simulink model "Path_Finder"  (R2024b)
settings: Solver=VariableStepAuto  StartTime=0.0  StopTime=200  RelTol=1e-3
model workspace (MAT data in the model file):
  Drag_Constants = 1
  mass = [5.51 5.51 5.51 1 1 1]
  mass_6a = [5 5 5 1 1 1]
libraries: simulink x1
settings Model: Creator=zenyn  LastModifiedBy=zenyn
settings DebuggingCC: UnderSpecifiedDimensionMsg=warning

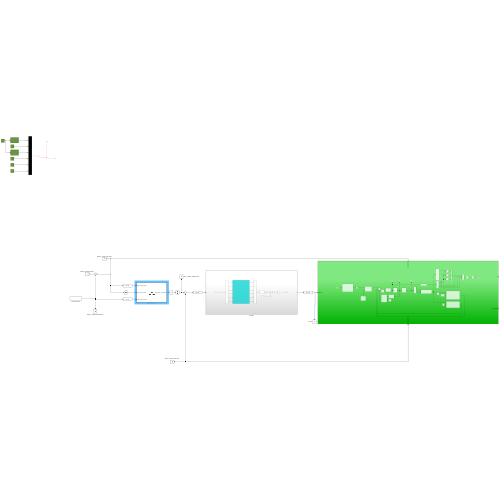
[thumbnail: Simulink's stored preview of the top-level diagram]
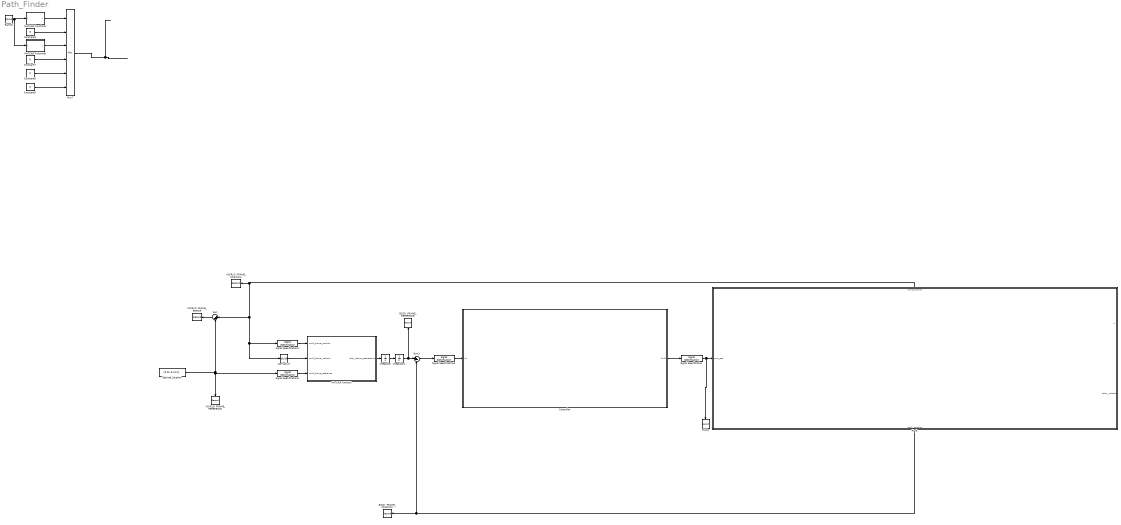
== system Path_Finder ==
  BODY_FRAME_POSITION : Record  FileSettingsInternal="{\"entries\":[{\"content\":{\"excelSettings\":{\"content\":{},\"type\":\"Streamout.ExcelSettings\"}},\"type\":\"Streamout.FileSettingStorage\",\"uuid\":\"\"}],\"packageUris\":[\"http:\\/\\/schema.mathworks.com\\/mf0\\/streamout_blocks\\/R2020a\"],\"version\":\"1.0\"}"  Layout=[1 1]  SignalsInternal="{\"entries\":[{\"content\":{},\"type\":\"RecordBlkView.InputSignals\",\"uuid\":\"\"}],\"packageUris\":[\"http:\\/\\/schema.mathworks.com\\/mf0\\/streamout_blocks\\/R2020a\"],\"version\":\"1.0\"}"  VisualizationBindings="{\"sparklinesplugin\":{\"info\":[{\"bindingParametersList\":[],\"subplotID\":1}]}}"
  BODY_FRAME_REFERENCE : Record  FileSettingsInternal="{\"entries\":[{\"content\":{\"excelSettings\":{\"content\":{},\"type\":\"Streamout.ExcelSettings\"}},\"type\":\"Streamout.FileSettingStorage\",\"uuid\":\"\"}],\"packageUris\":[\"http:\\/\\/schema.mathworks.com\\/mf0\\/streamout_blocks\\/R2020a\"],\"version\":\"1.0\"}"  SignalsInternal="{\"entries\":[{\"content\":{},\"type\":\"RecordBlkView.InputSignals\",\"uuid\":\"\"}],\"packageUris\":[\"http:\\/\\/schema.mathworks.com\\/mf0\\/streamout_blocks\\/R2020a\"],\"version\":\"1.0\"}"  VisualizationBindings="{\"sparklinesplugin\":{\"info\":[{\"bindingParametersList\":[],\"subplotID\":1}]}}"
  Constant{6..9} (4 alike) : Constant  Value=0
  Controller : Subsystem
  Derivative : Derivative
  Desired Location : Constant  Value=[0 20 -5 0 0 1]
  Integrator : Integrator
  Integrator1 : Integrator
  MATLAB Function : MATLAB Function  TreatAsAtomicUnit=on
  MATLAB Function6 : MATLAB Function  TreatAsAtomicUnit=on
  MATLAB Function8 : MATLAB Function  TreatAsAtomicUnit=on
  Mux7 : Mux  Inputs=6
  PWMs : Record  FileSettingsInternal="{\"entries\":[{\"content\":{\"excelSettings\":{\"content\":{},\"type\":\"Streamout.ExcelSettings\"}},\"type\":\"Streamout.FileSettingStorage\",\"uuid\":\"\"}],\"packageUris\":[\"http:\\/\\/schema.mathworks.com\\/mf0\\/streamout_blocks\\/R2020a\"],\"version\":\"1.0\"}"  Layout=[1 1]  SignalsInternal="{\"entries\":[{\"content\":{},\"type\":\"RecordBlkView.InputSignals\",\"uuid\":\"\"}],\"packageUris\":[\"http:\\/\\/schema.mathworks.com\\/mf0\\/streamout_blocks\\/R2020a\"],\"version\":\"1.0\"}"  VisualizationBindings="{\"sparklinesplugin\":{\"info\":[{\"bindingParametersList\":[],\"subplotID\":1}]}}"
  Plant : Subsystem
      settings: PortSchema="{\"entries\":[{\"content\":{\"sides\":[{\"content\":{\"connectorIds\":[\"In1\"]},\"type\":\"ConnectorPlacement.EquallySpacedRectSide\",\"uuid\":\"dd5f5d00-f9c2-4307-bbb7-eccecd8688a5\"},{\"content\":{\"connectorIds\":[\"Out1\",\"Out2\"],\"side\":\"RIGHT\"},\"type\":\"ConnectorPlacement.EquallySpacedRectSide\",\"uuid\":\"260bc773-df58-4a30-8a2b-ed16ecf586eb\"},{\"content\":{\"connectorIds\":[\"Out4\"],\"side\":\"TOP\"},\"type\":\"ConnectorPlacement.EquallySpacedRectSide\",\"uuid\":\"8636c4da-abe4-4bf1-a8cd-e88e3163142a\"},{\"content\":{\"connectorIds\":[\"Out3\"],\"side\":\"BOTTOM\"},\"type\":\"ConnectorPlacement.EquallySpacedRectSide\",\"uuid\":\"d94fc4d4-7054-443b-b127-f4054aef1378\"}]},\"type\":\"ConnectorPlacement.EquallySpacedConnector\",\"uuid\":\"031b742f-18b9-426f-a877-fafb44a51bf1\"}],\"packageUris\":[\"http://schema.mathworks.com/mf0/Connector/R2020b\"],\"version\":\"1.0\"}"
  Ramp2 : simulink/Sources/Ramp  slope=1  start=0  InitialOutput=0
  Signal Specification : SignalSpecification  Dimensions=[ 1 8]
  Signal Specification1 : SignalSpecification  Dimensions=[ 1 6]
  Signal Specification2 : SignalSpecification  Dimensions=[1 6]
  Signal Specification3 : SignalSpecification  Dimensions=[1 6]
  Sum : Sum  Inputs=|+-
  Sum1 : Sum  Inputs=|+-
  WORLD_FRAME_ERROR : Record  FileSettingsInternal="{\"entries\":[{\"content\":{\"excelSettings\":{\"content\":{},\"type\":\"Streamout.ExcelSettings\"}},\"type\":\"Streamout.FileSettingStorage\",\"uuid\":\"\"}],\"packageUris\":[\"http:\\/\\/schema.mathworks.com\\/mf0\\/streamout_blocks\\/R2020a\"],\"version\":\"1.0\"}"  Layout=[1 1]  SignalsInternal="{\"entries\":[{\"content\":{},\"type\":\"RecordBlkView.InputSignals\",\"uuid\":\"\"}],\"packageUris\":[\"http:\\/\\/schema.mathworks.com\\/mf0\\/streamout_blocks\\/R2020a\"],\"version\":\"1.0\"}"  VisualizationBindings="{\"sparklinesplugin\":{\"info\":[{\"bindingParametersList\":[],\"subplotID\":1}]}}"
  WORLD_FRAME_POSITION : Record  FileSettingsInternal="{\"entries\":[{\"content\":{\"excelSettings\":{\"content\":{},\"type\":\"Streamout.ExcelSettings\"}},\"type\":\"Streamout.FileSettingStorage\",\"uuid\":\"\"}],\"packageUris\":[\"http:\\/\\/schema.mathworks.com\\/mf0\\/streamout_blocks\\/R2020a\"],\"version\":\"1.0\"}"  Layout=[1 1]  SignalsInternal="{\"entries\":[{\"content\":{},\"type\":\"RecordBlkView.InputSignals\",\"uuid\":\"\"}],\"packageUris\":[\"http:\\/\\/schema.mathworks.com\\/mf0\\/streamout_blocks\\/R2020a\"],\"version\":\"1.0\"}"  VisualizationBindings="{\"sparklinesplugin\":{\"info\":[{\"bindingParametersList\":[],\"subplotID\":1}]}}"
  WORLD_FRAME_REFERENCE : Record  FileSettingsInternal="{\"entries\":[{\"content\":{\"excelSettings\":{\"content\":{},\"type\":\"Streamout.ExcelSettings\"}},\"type\":\"Streamout.FileSettingStorage\",\"uuid\":\"\"}],\"packageUris\":[\"http:\\/\\/schema.mathworks.com\\/mf0\\/streamout_blocks\\/R2020a\"],\"version\":\"1.0\"}"  Layout=[1 1]  SignalsInternal="{\"entries\":[{\"content\":{\"signals\":[{\"content\":{\"blockPath\":[],\"dimensions\":[1,6],\"domain\":\"\",\"hasChildren\":true,\"lineColor\":\"#edb120\",\"lineWidth\":2,\"port\":1,\"sid\":[\"\"],\"signalID\":1,\"signalName\":\"Plant:3\"},\"type\":\"RecordBlkView.Signal\",\"uuid\":\"\"},{\"content\":{\"blockPath\":[],\"channel\":[1,1],\"dimensions\":[1,6],\"domain\":\"\",\"lineColor\":\"#7e2f8e\",\"lineWidth\":2,\"parentID\":1,\"port\":1,\"sid\":[\"\"],\"signalID\":2,\"signalName\":\"Plant:3\"},\"type\":\"RecordBlkView.Signal\",\"uuid\":\"\"},{\"content\":{\"blockPath\":[],\"dimensions\":[1,6],\"domain\":\"\",\"hasChildren\":true,\"lineColor\":\"#77ac30\",\"lineWidth\":2,\"port\":1,\"sid\":[\"\"],\"signalID\":3,\"signalName\":\"Integrator1\"},\"type\":\"RecordBlkView.Signal\",\"uuid\":\"\"},{\"content\":{\"blockPath\":[],\"channel\":[1,1],\"dimensions\":[1,6],\"domain\":\"\",\"lineColor\":\"#0072bd\",\"lineWidth\":2,\"parentID\":3,\"port\":1,\"sid\":[\"\"],\"signalID\":4,\"signalName\":\"Integrator1\"},\"type\":\"RecordBlkView.Signal\",\"uuid\":\"\"},{\"content\":{\"blockPath\":[],\"dimensions\":[1,8],\"domain\":\"\",\"hasChildren\":true,\"lineColor\":\"#a2142f\",\"lineWidth\":2,\"port\":1,\"sid\":[\"\"],\"signalID\":5,\"signalName\":\"Signal Specification\"},\"type\":\"RecordBlkView.Signal\",\"uuid\":\"\"},{\"content\":{\"blockPath\":[],\"channel\":[1,1],\"dimensions\":[1,8],\"domain\":\"\",\"lineColor\":\"#139fff\",\"lineWidth\":2,\"parentID\":5,\"port\":1,\"sid\":[\"\"],\"signalID\":6,\"signalName\":\"Signal Specification\"},\"type\":\"RecordBlkView.Signal\",\"uuid\":\"\"},{\"content\":{\"blockPath\":[],\"dimensions\":[6],\"domain\":\"\",\"hasChildren\":true,\"lineColor\":\"#ff6929\",\"lineWidth\":2,\"port\":1,\"sid\":[\"\"],\"signalID\":7,\"signalName\":\"Sum\"},\"type\":\"RecordBlkView.Signal\",\"uuid\":\"\"},{\"content\":{\"blockPath\":[],\"channel\":[1],\"dimensions\":[6],\"domain\":\"\",\"lineColor\":\"#edb120\",\"lineWidth\":2,\"parentID\":7,\"port\":1,\"sid\":[\"\"],\"signalID\":8,\"signalName\":\"Sum\"},\"type\":\"RecordBlkView.Signal\",\"uuid\":\"\"},{\"content\":{\"blockPath\":[],\"dimensions\":[6],\"domain\":\"\",\"hasChildren\":true,\"lineColor\":\"#64d413\",\"lineWidth\":2,\"port\":1,\"sid\":[\"\"],\"signalID\":9,\"signalName\":\"Plant:4\"},\"type\":\"RecordBlkView.Signal\",\"uuid\":\"\"},{\"content\":{\"blockPath\":[],\"channel\":[1],\"dimensions\":[6],\"domain\":\"\",\"lineColor\":\"#ff13a6\",\"lineWidth\":2,\"parentID\":9,\"port\":1,\"sid\":[\"\"],\"signalID\":10,\"signalName\":\"Plant:4\"},\"type\":\"RecordBlkView.Signal\",\"uuid\":\"\"},{\"content\":{\"blockPath\":[],\"dimensions\":[1,6],\"domain\":\"\",\"hasChildren\":true,\"lineColor\":\"#fe330a\",\"lineWidth\":2,\"port\":1,\"sid\":[\"\"],\"signalID\":11},\"type\":\"RecordBlkView.Signal\",\"uuid\":\"\"},{\"content\":{\"blockPath\":[],\"channel\":[1,1],\"dimensions\":[1,6],\"domain\":\"\",\"lineColor\":\"#22b573\",\"lineWidth\":2,\"parentID\":11,\"port\":1,\"sid\":[\"\"],\"signalID\":12},\"type\":\"RecordBlkView.Signal\",\"uuid\":\"\"},{\"content\":{\"blockPath\":[],\"dimensions\":[6],\"domain\":\"\",\"hasChildren\":true,\"lineColor\":\"#0072bd\",\"lineWidth\":2,\"port\":1,\"sid\":[\"\"],\"signalID\":13,\"signalName\":\"Desired Location\"},\"type\":\"RecordBlkView.Signal\",\"uuid\":\"\"},{\"content\":{\"blockPath\":[],\"channel\":[1],\"dimensions\":[6],\"domain\":\"\",\"lineColor\":\"#d95319\",\"lineWidth\":2,\"parentID\":13,\"port\":1,\"sid\":[\"\"],\"signalID\":14,\"signalName\":\"Desired Location\"},\"type\":\"RecordBlkView.Signal\",\"uuid\":\"\"},{\"content\":{\"blockPath\":[],\"channel\":[2],\"dimensions\":[6],\"domain\":\"\",\"lineColor\":\"#a2142f\",\"lineWidth\":2,\"parentID\":7,\"port\":1,\"sid\":[\"\"],\"signalID\":15,\"signalName\":\"Sum\"},\"type\":\"RecordBlkView.Signal\",\"uuid\":\"\"},{\"content\":{\"blockPath\":[],\"channel\":[3],\"dimensions\":[6],\"domain\":\"\",\"lineColor\":\"#139fff\",\"lineWidth\":2,\"parentID\":7,\"port\":1,\"sid\":[\"\"],\"signalID\":16,\"signalName\":\"Sum\"},\"type\":\"RecordBlkView.Signal\",\"uuid\":\"\"},{\"content\":{\"blockPath\":[],\"channel\":[4],\"dimensions\":[6],\"domain\":\"\",\"lineColor\":\"#ff6929\",\"lineWidth\":2,\"parentID\":7,\"port\":1,\"sid\":[\"\"],\"signalID\":17,\"signalName\":\"Sum\"},\"type\":\"RecordBlkView.Signal\",\"uuid\":\"\"},{\"content\":{\"blockPath\":[],\"channel\":[5],\"dimensions\":[6],\"domain\":\"\",\"lineColor\":\"#b746ff\",\"lineWidth\":2,\"parentID\":7,\"port\":1,\"sid\":[\"\"],\"signalID\":18,\"signalName\":\"Sum\"},\"type\":\"RecordBlkView.Signal\",\"uuid\":\"\"},{\"content\":{\"blockPath\":[],\"channel\":[6],\"dimensions\":[6],\"domain\":\"\",\"lineColor\":\"#64d413\",\"lineWidth\":2,\"parentID\":7,\"port\":1,\"sid\":[\"\"],\"signalID\":19,\"signalName\":\"Sum\"},\"type\":\"RecordBlkView.Signal\",\"uuid\":\"\"},{\"content\":{\"blockPath\":[],\"channel\":[1,2],\"dimensions\":[1,6],\"domain\":\"\",\"lineColor\":\"#139fff\",\"lineWidth\":2,\"parentID\":3,\"port\":1,\"sid\":[\"\"],\"signalID\":20,\"signalName\":\"Integrator1\"},\"type\":\"RecordBlkView.Signal\",\"uuid\":\"\"},{\"content\":{\"blockPath\":[],\"channel\":[1,3],\"dimensions\":[1,6],\"domain\":\"\",\"lineColor\":\"#ff6929\",\"lineWidth\":2,\"parentID\":3,\"port\":1,\"sid\":[\"\"],\"signalID\":21,\"signalName\":\"Integrator1\"},\"type\":\"RecordBlkView.Signal\",\"uuid\":\"\"},{\"content\":{\"blockPath\":[],\"channel\":[1,4],\"dimensions\":[1,6],\"domain\":\"\",\"lineColor\":\"#b746ff\",\"lineWidth\":2,\"parentID\":3,\"port\":1,\"sid\":[\"\"],\"signalID\":22,\"signalName\":\"Integrator1\"},\"type\":\"RecordBlkView.Signal\",\"uuid\":\"\"},{\"content\":{\"blockPath\":[],\"channel\":[1,5],\"dimensions\":[1,6],\"domain\":\"\",\"lineColor\":\"#64d413\",\"lineWidth\":2,\"parentID\":3,\"port\":1,\"sid\":[\"\"],\"signalID\":23,\"signalName\":\"Integrator1\"},\"type\":\"RecordBlkView.Signal\",\"uuid\":\"\"},{\"content\":{\"blockPath\":[],\"channel\":[1,6],\"dimensions\":[1,6],\"domain\":\"\",\"lineColor\":\"#ff13a6\",\"lineWidth\":2,\"parentID\":3,\"port\":1,\"sid\":[\"\"],\"signalID\":24,\"signalName\":\"Integrator1\"},\"type\":\"RecordBlkView.Signal\",\"uuid\":\"\"}]},\"type\":\"RecordBlkView.InputSignals\",\"uuid\":\"\"}],\"packageUris\":[\"http:\\/\\/schema.mathworks.com\\/mf0\\/streamout_blocks\\/R2020a\"],\"version\":\"1.0\"}"  VisualizationBindings="{\"sparklinesplugin\":{\"info\":[{\"bindingParametersList\":[],\"subplotID\":1}]}}"
  wires:
  Plant/4(world_position) -> Sum/1, Derivative/1, Signal Specification1/1, WORLD_FRAME_POSITION/1
  MATLAB Function8/1(y) -> Mux7/3
  Mux7/1 -> ?
  Constant6/1 -> Mux7/2
  Ramp2/1 -> MATLAB Function6/1(t), MATLAB Function8/1(t)
  Constant8/1 -> Mux7/5
  Constant9/1 -> Mux7/6
  MATLAB Function6/1(y) -> Mux7/1
  Constant7/1 -> Mux7/4
  Desired Location/1 -> Sum/2, Signal Specification2/1, WORLD_FRAME_REFERENCE/1
  Controller/1(Out1) -> Signal Specification/1
  Signal Specification/1 -> PWMs/1, Plant/1(pwm_set)
  Plant/3(body_position) -> Sum1/2, BODY_FRAME_POSITION/1
  Signal Specification3/1 -> Controller/1(In1)
  Sum1/1 -> Signal Specification3/1
  Signal Specification1/1 -> MATLAB Function/1(world_frame_position)
  Signal Specification2/1 -> MATLAB Function/3(world_frame_reference)
  MATLAB Function/1(body_frame_acceleration) -> Integrator/1
  Integrator/1 -> Integrator1/1
  Sum/1 -> WORLD_FRAME_ERROR/1
  Derivative/1 -> MATLAB Function/2(world_frame_velocity)
  Integrator1/1 -> BODY_FRAME_REFERENCE/1, Sum1/1

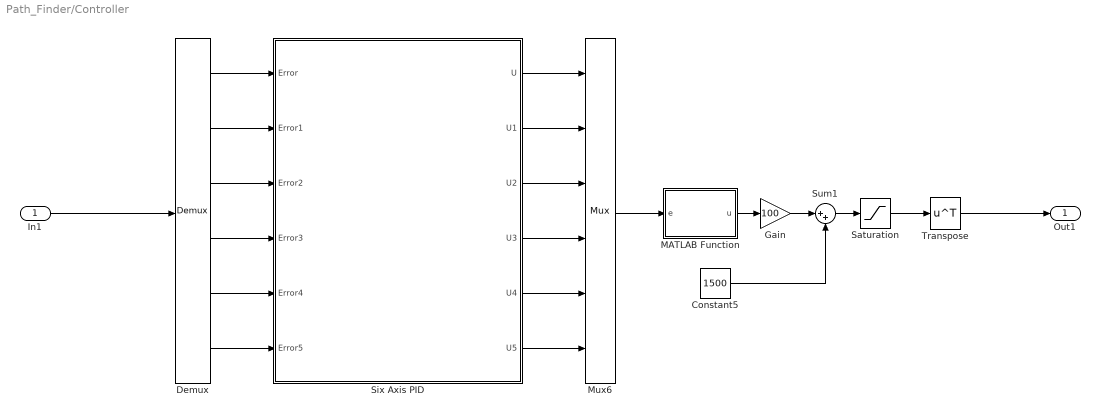
== system Path_Finder/Controller ==
  In1 : Inport
  Constant5 : Constant  Value=1500
  Demux : Demux  Outputs=6
  Gain : Gain  Gain=100
  MATLAB Function : MATLAB Function  TreatAsAtomicUnit=on
  Mux6 : Mux  Inputs=6
  Saturation : Saturate  UpperLimit=1900  LowerLimit=1100
  Six Axis PID : Subsystem
  Sum1 : Sum  Inputs=|++
  Transpose : Math  Operator=transpose
  Out1 : Outport
  wires:
  Saturation/1 -> Transpose/1
  Sum1/1 -> Saturation/1
  Demux/6 -> Six Axis PID/6(Error5)
  MATLAB Function/1(u) -> Gain/1
  Demux/3 -> Six Axis PID/3(Error2)
  In1/1 -> Demux/1
  Demux/5 -> Six Axis PID/5(Error4)
  Constant5/1 -> Sum1/2
  Demux/4 -> Six Axis PID/4(Error3)
  Demux/2 -> Six Axis PID/2(Error1)
  Demux/1 -> Six Axis PID/1(Error)
  Transpose/1 -> Out1/1
  Six Axis PID/3(U2) -> Mux6/3
  Gain/1 -> Sum1/1
  Six Axis PID/1(U) -> Mux6/1
  Six Axis PID/2(U1) -> Mux6/2
  Six Axis PID/4(U3) -> Mux6/4
  Six Axis PID/5(U4) -> Mux6/5
  Six Axis PID/6(U5) -> Mux6/6
  Mux6/1 -> MATLAB Function/1(e)

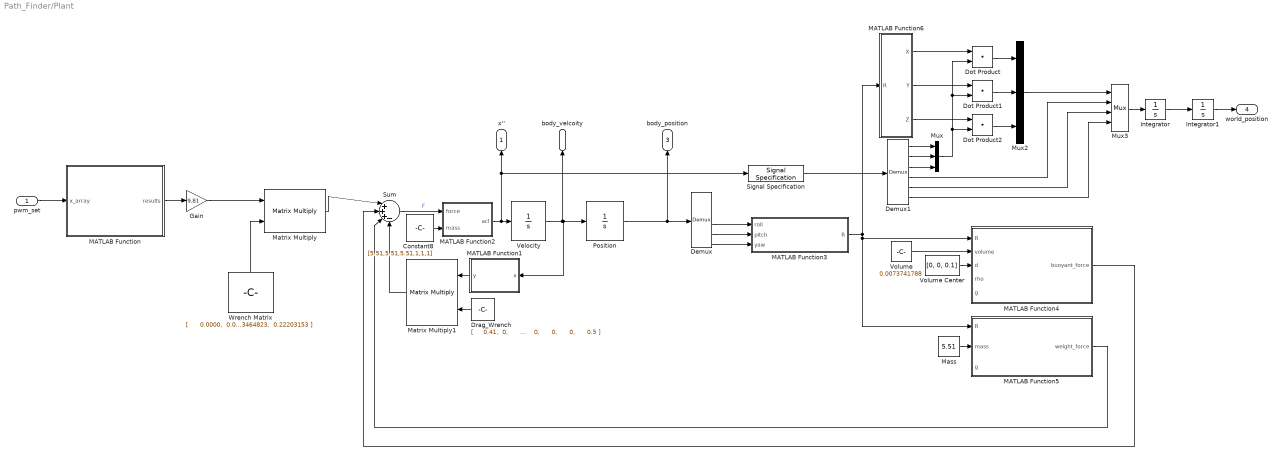
== system Path_Finder/Plant ==
  pwm_set : Inport
  Constant8 : Constant  Value=[5.51,5.51,5.51,1,1,1]  VectorParams1D=off
  Demux : Demux  Outputs=6
  Demux1 : Demux  Outputs=6
  Dot Product : DotProduct  OutDataTypeStr=Inherit: Inherit via internal rule
  Dot Product1 : DotProduct  OutDataTypeStr=Inherit: Inherit via internal rule
  Dot Product2 : DotProduct  OutDataTypeStr=Inherit: Inherit via internal rule
  Drag_Wrench : Constant  Value=|  VectorParams1D=off
      | [
      |     0.41,  0,      0,      0,      0,      0;
      |     0,      0.5,   0,      0,      0,      0;
      |     0,      0,      1.25,  0,      0,      0;
      |     0,      0,      0,      0.5,   0,      0;
      |     0,      0,      0,      0,      1,    0;
      |     0,      0,      0,      0,      0,      0.5
      | ]
  Gain : Gain  Gain=9.81
  Integrator : Integrator
  Integrator1 : Integrator
  MATLAB Function : MATLAB Function  TreatAsAtomicUnit=on
  MATLAB Function1 : MATLAB Function  TreatAsAtomicUnit=on
  MATLAB Function2 : MATLAB Function  TreatAsAtomicUnit=on
  MATLAB Function3 : MATLAB Function  TreatAsAtomicUnit=on
  MATLAB Function4 : MATLAB Function  TreatAsAtomicUnit=on
  MATLAB Function5 : MATLAB Function  TreatAsAtomicUnit=on
  MATLAB Function6 : MATLAB Function  TreatAsAtomicUnit=on
  Mass : Constant  Value=5.51
  Matrix Multiply : Product  Multiplication=Matrix(*)
  Matrix Multiply1 : Product  Multiplication=Matrix(*)
  Mux : Mux  Inputs=3
  Mux2 : Mux  Inputs=3
  Mux3 : Mux
  Position : Integrator
  Signal Specification : SignalSpecification  Dimensions=[1 6]
  Sum : Sum  Inputs=|+++-
  Velocity : Integrator
  Volume : Constant  Value=0.0073741788
  Volume Center : Constant  Value=[0, 0, 0.1]
  Wrench Matrix : Constant  Value=|  VectorParams1D=off
      | [
      |      0.0000,  0.0000,  1.0000, -0.2035, -0.2535,  0.0000;
      |      0.0000,  0.0000,  1.0000,  0.2035, -0.2535,  0.0000;
      |      0.0000,  0.0000,  1.0000, -0.2035,  0.2545,  0.0000;
      |      0.0000,  0.0000,  1.0000,  0.2035,  0.2545,  0.0000;
      |     -0.7071, -0.7071,  0.0000, -0.03464823,  0.03464823, -0.21531401;
      |     -0.7071,  0.7071,  0.0000,  0.03464823,  0.03464823,  0.21531401;
      |     -0.7071,  0.7071,  0.0000,  0.03464823,  0.03464823, -0.22203153;
      |     -0.7071, -0.7071,  0.0000, -0.03464823,  0.03464823,  0.22203153
      | ]
  x'' : Outport
  body_velcoity : Outport  Port=2
  body_position : Outport  Port=3
  world_position : Outport  Port=4
  wires:
  Demux/4 -> MATLAB Function3/1(roll)
  Volume/1 -> MATLAB Function4/2(volume)
  Volume Center/1 -> MATLAB Function4/3(d)
  Sum/1 -> MATLAB Function2/1(force)  "F"
  Drag_Wrench/1 -> Matrix Multiply1/2
  Demux/6 -> MATLAB Function3/3(yaw)
  MATLAB Function1/1(y) -> Matrix Multiply1/1
  MATLAB Function5/1(weight_force) -> Sum/3
  Constant8/1 -> MATLAB Function2/2(mass)
  Velocity/1 -> Position/1, MATLAB Function1/1(x), body_velcoity/1
  MATLAB Function/1(results) -> Gain/1
  Mass/1 -> MATLAB Function5/2(mass)
  Position/1 -> body_position/1, Demux/1
  Wrench Matrix/1 -> Matrix Multiply/2
  MATLAB Function3/1(R) -> MATLAB Function5/1(R), MATLAB Function4/1(R), MATLAB Function6/1(R)
  MATLAB Function2/1(acl) -> Signal Specification/1, x''/1, Velocity/1
  Demux/5 -> MATLAB Function3/2(pitch)
  Matrix Multiply1/1 -> Sum/4
  pwm_set/1 -> MATLAB Function/1(x_array)
  Integrator/1 -> Integrator1/1
  Matrix Multiply/1 -> Sum/1
  MATLAB Function4/1(buoyant_force) -> Sum/2
  Gain/1 -> Matrix Multiply/1
  Signal Specification/1 -> Demux1/1
  Demux1/3 -> Mux/3
  Demux1/2 -> Mux/2
  Demux1/1 -> Mux/1
  Mux/1 -> Dot Product2/2, Dot Product1/2, Dot Product/2
  MATLAB Function6/1(X) -> Dot Product/1
  MATLAB Function6/2(Y) -> Dot Product1/1
  MATLAB Function6/3(Z) -> Dot Product2/1
  Dot Product/1 -> Mux2/1
  Dot Product1/1 -> Mux2/2
  Dot Product2/1 -> Mux2/3
  Mux2/1 -> Mux3/1
  Demux1/4 -> Mux3/2
  Mux3/1 -> Integrator/1
  Demux1/5 -> Mux3/3
  Demux1/6 -> Mux3/4
  Integrator1/1 -> world_position/1

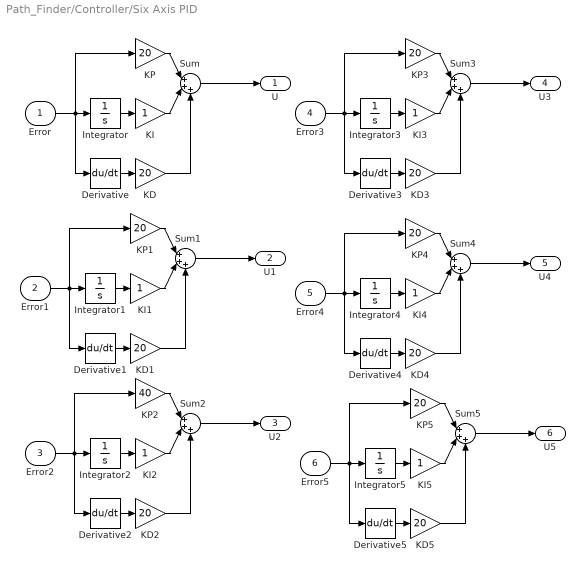
== system Path_Finder/Controller/Six Axis PID ==
  Error : Inport
  Error1 : Inport  Port=2
  Error2 : Inport  Port=3
  Error3 : Inport  Port=4
  Error4 : Inport  Port=5
  Error5 : Inport  Port=6
  Derivative{,1..5} (6 alike) : Derivative
  Integrator{,1..5} (6 alike) : Integrator
  KD{,1..5} (6 alike) : Gain  Gain=20
  KI{,1..5} (6 alike) : Gain
  KP{,1,3..5} (5 alike) : Gain  Gain=20
  KP2 : Gain  Gain=40
  Sum{,1..5} (6 alike) : Sum  Inputs=|+++
  U : Outport
  U1 : Outport  Port=2
  U2 : Outport  Port=3
  U3 : Outport  Port=4
  U4 : Outport  Port=5
  U5 : Outport  Port=6
  wires:
  Integrator4/1 -> KI4/1
  Sum3/1 -> U3/1
  KI4/1 -> Sum4/2
  KP1/1 -> Sum1/1
  Integrator5/1 -> KI5/1
  Derivative/1 -> KD/1
  KD5/1 -> Sum5/3
  KD4/1 -> Sum4/3
  Derivative5/1 -> KD5/1
  Derivative2/1 -> KD2/1
  KI1/1 -> Sum1/2
  Integrator/1 -> KI/1
  KD/1 -> Sum/3
  KD2/1 -> Sum2/3
  Derivative3/1 -> KD3/1
  Error3/1 -> Derivative3/1, Integrator3/1, KP3/1
  KI5/1 -> Sum5/2
  KI3/1 -> Sum3/2
  KI/1 -> Sum/2
  Error5/1 -> Derivative5/1, Integrator5/1, KP5/1
  Integrator1/1 -> KI1/1
  Error/1 -> KP/1, Derivative/1, Integrator/1
  KD3/1 -> Sum3/3
  KI2/1 -> Sum2/2
  Integrator3/1 -> KI3/1
  Error2/1 -> Derivative2/1, Integrator2/1, KP2/1
  KP2/1 -> Sum2/1
  Integrator2/1 -> KI2/1
  KP4/1 -> Sum4/1
  Derivative1/1 -> KD1/1
  KD1/1 -> Sum1/3
  Error4/1 -> Derivative4/1, Integrator4/1, KP4/1
  KP3/1 -> Sum3/1
  KP/1 -> Sum/1
  KP5/1 -> Sum5/1
  Sum2/1 -> U2/1
  Sum/1 -> U/1
  Sum4/1 -> U4/1
  Sum5/1 -> U5/1
  Derivative4/1 -> KD4/1
  Sum1/1 -> U1/1
  Error1/1 -> Derivative1/1, Integrator1/1, KP1/1

== matlab function Path_Finder/Plant/MATLAB Function1 ==
  data: x input; y output
function y = signed_square(x)
y = x .* abs(x);
end

== matlab function Path_Finder/Plant/MATLAB Function ==
  data: x_array input; results output
function results = pwm_function(x_array)
    % Preallocate results array
    results = zeros(size(x_array)); 
    
    % First condition: 1100 <= x < 1460
    idx = (x_array >= 1100 & x_array < 1460);
    results(idx) = (-1.24422882971549e-8) * x_array(idx).^3 ...
                 + (4.02057100632393e-5) * x_array(idx).^2 ...
                 - 0.0348619861030835 * x_array(idx) ...
                 + 3.90671429105423;
    
    % Second condition: 1460 <= x <= 1540
    idx = (x_array >= 1460 & x_array <= 1540);
    results(idx) = 0;
    
    % Third condition: 1540 < x <= 1900
    idx = (x_array > 1540 & x_array <= 1900);
    results(idx) = (-1.64293565374284e-8) * x_array(idx).^3 ...
                 + (9.45962838560648e-5) * x_array(idx).^2 ...
                 - 0.170812079190679 * x_array(idx) ...
                 + 98.7232373648272;
    
    % Handle out-of-range values
    if any(isnan(results))
        error('Some values in x_array are out of the valid range [1100..1900].');
    end
end

== matlab function Path_Finder/Plant/MATLAB Function2 ==
  data: force input; acl output; mass input
function acl = fcn(force, mass)
acl = force ./ mass;

end

== matlab function Path_Finder/Plant/MATLAB Function3 ==
  data: roll input; R output; pitch input; yaw input
function R = rotation_matrix(roll, pitch, yaw)
    % Rotation matrix around X-axis (roll)
    Rx = [
        1,  0,           0;
        0,  cos(roll),  -sin(roll);
        0,  sin(roll),   cos(roll)
    ];

    % Rotation matrix around Y-axis (pitch)
    Ry = [
        cos(pitch),  0,  sin(pitch);
        0,           1,  0;
       -sin(pitch),  0,  cos(pitch)
    ];

    % Rotation matrix around Z-axis (yaw)
    Rz = [
        cos(yaw), -sin(yaw),  0;
        sin(yaw),  cos(yaw),  0;
        0,         0,         1
    ];

    % Combine rotations: R = Rz * Ry * Rx
    R = Rz * Ry * Rx;
end

== matlab function Path_Finder/Plant/MATLAB Function4 ==
  data: R input; buoyant_force output; volume input; d input; rho input; g input
function buoyant_force = buoyant_force(R, volume, d, rho, g)
    % Set default values for fluid density and gravity if not provided
    if nargin < 6
        rho = 1000; % Default fluid density (kg/m³) for water
    end
    if nargin < 7
        g = 9.81; % Default gravitational acceleration (m/s²)
    end

    % Ensure d is a column vector
    d = d(:);

    % Buoyant force vector in world frame
    b_vector = [0; 0; rho * g * volume];

    % Rotate buoyant force to object's frame
    buoyant_force_body = R * b_vector;

    % Compute torque using cross product τ = d × F_buoyancy
    % (MATLAB cross function works for column vectors)
    torque = cross(-d, buoyant_force_body);

    % Combine force and torque into a single output vector
    buoyant_force = [buoyant_force_body; torque]';
end

== matlab function Path_Finder/Plant/MATLAB Function5 ==
  data: R input; weight_force output; mass input; g input
function weight_force = weight_force(R, mass, g)
    % Set default gravitational acceleration if not provided
    if nargin < 4
        g = 9.81; % Default gravitational acceleration (m/s²)
    end

    % Gravity force vector in world frame (downward)
    g_vector = [0; 0; -mass * g];
    
    % Linear Force
    lin = R * g_vector;
    % Rotational force
    rot = [0;0;0];
    % Transform gravity force to rotated frame
    weight_force = [lin', rot'];
end

== matlab function Path_Finder/MATLAB Function6 ==
  data: t input; y output
function y = fcn(t)

if t < 30
    y = t;
elseif t < 60
    y = 30;
else
    y = 90 - t;

end

== matlab function Path_Finder/Controller/MATLAB Function ==
  data: e input; u output
function u = rev_wrench(e)

wrench_matrix = [
     0.0000,  0.0000,  1.0000, -0.2035, -0.2535,  0.0000;
     0.0000,  0.0000,  1.0000,  0.2035, -0.2535,  0.0000;
     0.0000,  0.0000,  1.0000, -0.2035,  0.2545,  0.0000;
     0.0000,  0.0000,  1.0000,  0.2035,  0.2545,  0.0000;
    -0.7071, -0.7071,  0.0000, -0.03464823,  0.03464823, -0.21531401;
    -0.7071,  0.7071,  0.0000,  0.03464823,  0.03464823,  0.21531401;
    -0.7071,  0.7071,  0.0000,  0.03464823,  0.03464823, -0.22203153;
    -0.7071, -0.7071,  0.0000, -0.03464823,  0.03464823,  0.22203153];

inv_wrench = pinv(wrench_matrix);

u = inv_wrench' * e;
end

== matlab function Path_Finder/Plant/MATLAB Function6 ==
  data: R input; X output; Y output; Z output
function [X, Y, Z] =  axes(R)
% in this function, x, y and z axes refer to direction relative current
% orientation of robot

% X, Y and Z axes refer to direction relative to intial orientation of
% robot

x_vector = [1; 0; 0];
y_vector = [0; 1; 0];
z_vector = [0; 0; 1];

X = [R * x_vector];
Y = [R * y_vector];
Z = [R * z_vector];

end

== matlab function Path_Finder/MATLAB Function8 ==
  data: t input; y output
function y = fcn(t)

speed = 30 / 30; 
if t < 30
    y = 0;
elseif t < 60
    y = 30 * speed - t * speed;
else
    y = 30 * speed - 60 * speed;
end

== matlab function Path_Finder/MATLAB Function ==
  data: world_frame_position input; world_frame_velocity input; body_frame_acceleration output; world_frame_reference input
function body_frame_acceleration = path_finder( ...
    world_frame_position, ...
    world_frame_velocity, ...
    world_frame_reference)
    
    body_frame_acceleration = [0 0 0 0 0 0 ];

end
